simulink model "LinuxMPC"  (Simulink 7.9)
settings: Solver=ode45  StartTime=0.0  StopTime=60  RelTol=1e-3
values from neighbouring files (symbols this model uses):
  P_0 = eye(8)*100    [MPC_setup.m]
  R1 = sqrtm(R)    [MPC_setup.m]
  Ts_control = 0.02    [MPC_setup.m]
  Ts_kalman = 0.01    [MPC_setup.m]
  x_0 = [0,-pi/4,0,0,0,0,0,0]    [MPC_setup.m]
libraries: simulink x3
settings Model: Creator=tna13skn  LastModifiedBy=tna13skn

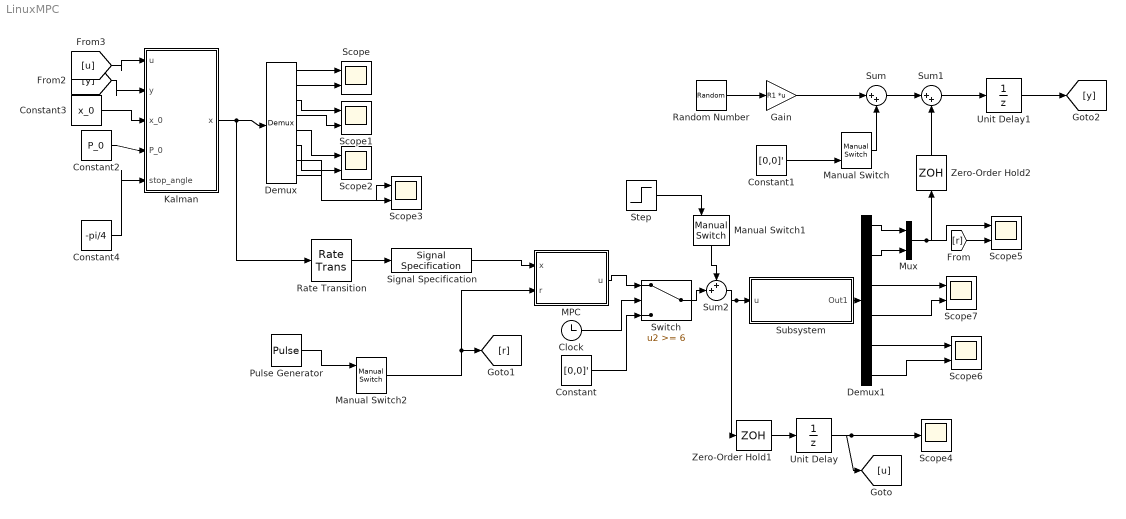
== system LinuxMPC ==
  Clock : Clock
  Constant : Constant  Value=[0,0]'
  Constant1 : Constant  Value=[0,0]'
  Constant2 : Constant  Value=P_0  VectorParams1D=off  SampleTime=Ts_kalman
  Constant3 : Constant  Value=x_0  SampleTime=Ts_kalman
  Constant4 : Constant  Value=-pi/4  SampleTime=Ts_kalman
  Demux : Demux  Outputs=8
  Demux1 : Demux  Outputs=6
  Gain : Gain  Gain=R1  Multiplication=Matrix(K*u)
  Kalman : MATLAB Function  TreatAsAtomicUnit=on
  MPC : MATLAB Function  TreatAsAtomicUnit=on
  Manual Switch : simulink/Signal Routing/Manual Switch  sw=1  action=0  varsize=off
  Manual Switch1 : simulink/Signal Routing/Manual Switch  sw=0  action=0  varsize=off
  Manual Switch2 : simulink/Signal Routing/Manual Switch  sw=1  action=0  varsize=off
  Mux : Mux  Inputs=2
  Pulse Generator : DiscretePulseGenerator  Amplitude=[0,-pi/7]'  Period=20/Ts_control  PulseWidth=10/Ts_control  SampleTime=Ts_control
  Random Number : RandomNumber  Mean=[0,0]'  Variance=[1,1]'  Seed=[1,3]  SampleTime=Ts_kalman
  Rate Transition : RateTransition  X0=x_0  OutPortSampleTime=Ts_control
  Scope{,1..3,5..7} (7 alike) : Scope  NumInputPorts=2
      Scope settings: YMin=-5~-5  YMax=5~5
      Scope1 settings: YMin=-5~-5  YMax=5~5
      Scope2 settings: YMin=-5~-5  YMax=5~5  SaveName=ScopeData2
      Scope3 settings: YMin=-5~-5  YMax=5~5  SaveName=ScopeData3
      Scope5 settings: YMin=-0.8~-0.45  YMax=0.1~0  SaveName=ScopeData5
      Scope6 settings: YMin=-5~-5  YMax=5~5  SaveName=ScopeData6
      Scope7 settings: YMin=-5~-5  YMax=5~5  SaveName=ScopeData7
  Scope4 : Scope
      settings: SaveName=ScopeData4
  Signal Specification : SignalSpecification  Dimensions=[8,1]  SampleTime=Ts_control
      settings: LockScale=on
  Step : Step  Time=30  Before=[0,0]'  After=[1,1]'*0.3  SampleTime=0
  Subsystem : Subsystem
  Sum : Sum  Inputs=|++
  Sum1 : Sum  Inputs=|++
  Sum2 : Sum  Inputs=++|
  Switch : Switch  Threshold=6
  Unit Delay : UnitDelay  SampleTime=-1
  Unit Delay1 : UnitDelay  SampleTime=-1
  Zero-Order Hold1 : ZeroOrderHold  SampleTime=Ts_kalman
  Zero-Order Hold2 : ZeroOrderHold  SampleTime=Ts_kalman
  wires:
  Kalman/1(x) -> Demux/1, Rate Transition/1
  Demux/1 -> Scope/1
  Demux/2 -> Scope/2
  Demux/3 -> Scope1/1
  Demux/4 -> Scope1/2
  Demux/5 -> Scope2/1
  Demux/6 -> Scope2/2
  Rate Transition/1 -> Signal Specification/1
  Signal Specification/1 -> MPC/1(x)
  MPC/1(u) -> Switch/1
  Clock/1 -> Switch/2
  Constant/1 -> Switch/3
  Subsystem/1(Out1) -> Demux1/1
  Demux/7 -> Scope3/1
  Demux/8 -> Scope3/2
  Zero-Order Hold1/1 -> Unit Delay/1
  Unit Delay/1 -> Scope4/1, [u]
  Demux1/1 -> Mux/1
  Demux1/2 -> Mux/2
  Mux/1 -> Scope5/1, Zero-Order Hold2/1
  [r] -> Scope5/2
  Demux1/3 -> Scope7/1
  Demux1/4 -> Scope7/2
  Demux1/5 -> Scope6/1
  Demux1/6 -> Scope6/2
  Random Number/1 -> Gain/1
  Constant1/1 -> Manual Switch/2
  Gain/1 -> Sum/1
  Manual Switch/1 -> Sum/2
  Sum1/1 -> Unit Delay1/1
  Sum/1 -> Sum1/1
  Zero-Order Hold2/1 -> Sum1/2
  Sum2/1 -> Subsystem/1(u), Zero-Order Hold1/1
  Manual Switch1/1 -> Sum2/1
  Step/1 -> Manual Switch1/1
  Manual Switch2/1 -> MPC/2(r), [r]
  Unit Delay1/1 -> [y]
  Pulse Generator/1 -> Manual Switch2/1
  Constant2/1 -> Kalman/4(P_0)
  Constant3/1 -> Kalman/3(x_0)
  [y] -> Kalman/2(y)
  [u] -> Kalman/1(u)
  Constant4/1 -> Kalman/5(stop_angle)
  Switch/1 -> Sum2/2

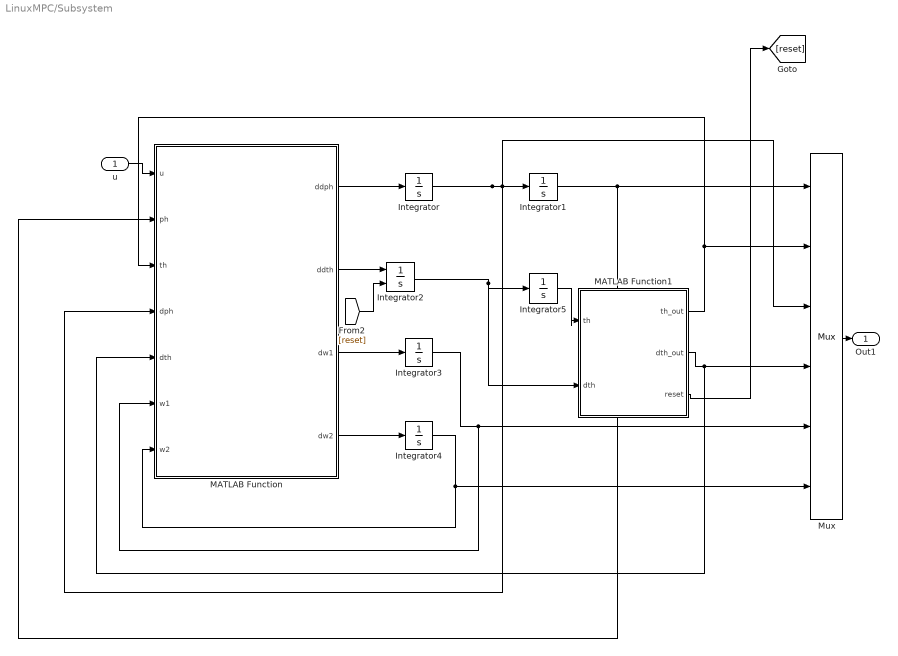
== system LinuxMPC/Subsystem ==
  u : Inport
  Integrator{,1,3..4} (4 alike) : Integrator
  Integrator2 : Integrator  ExternalReset=rising  ShowStatePort=on
  Integrator5 : Integrator  ShowStatePort=on
  MATLAB Function : MATLAB Function  TreatAsAtomicUnit=on
  MATLAB Function1 : MATLAB Function  TreatAsAtomicUnit=on
  Mux : Mux  Inputs=6
  Out1 : Outport
  wires:
  u/1 -> MATLAB Function/1(u)
  MATLAB Function/1(ddph) -> Integrator/1
  Integrator/1 -> Integrator1/1, MATLAB Function/4(dph), Mux/3
  Integrator1/1 -> Mux/1, MATLAB Function/2(ph)
  Mux/1 -> Out1/1
  MATLAB Function/2(ddth) -> Integrator2/1
  MATLAB Function/3(dw1) -> Integrator3/1
  MATLAB Function/4(dw2) -> Integrator4/1
  Integrator4/1 -> Mux/6, MATLAB Function/7(w2)
  Integrator3/1 -> Mux/5, MATLAB Function/6(w1)
  [reset] -> Integrator2/2
  MATLAB Function1/1(th_out) -> Mux/2, MATLAB Function/3(th)
  MATLAB Function1/2(dth_out) -> Mux/4, MATLAB Function/5(dth)
  Integrator5/1 -> MATLAB Function1/1(th)
  Integrator2/1 -> MATLAB Function1/2(dth), Integrator5/1
  MATLAB Function1/3(reset) -> [reset]

== matlab function MPC ==
  data: u output double; x input double; r input double
function u = MPC(x,r)
coder.extrinsic('mycsolve');
u=[0;0];
u=mycsolve(x,r);
end

== matlab function Kalman ==
  data: u input double; y input double; x_0 input double; P_0 input double; stop_angle input double; x output double
function x = kalman(u,y,x_0,P_0,stop_angle)

persistent x_hat;
persistent P;
if(isempty(x_hat))
    x_hat=x_0;
    P=P_0;
end
coder.extrinsic('updateKalman');

[x_hat,P]=updateKalman(x_hat,u,y,P,stop_angle);

x=x_hat;

== matlab function Subsystem/MATLAB Function ==
  data: u input double; ddph output double; ph input double; th input double; dph input double; dth input double; w1 input double; w2 input double; ddth output double; dw1 output double; dw2 output double
function [ddph, ddth, dw1, dw2] = fcn(u, ph, th, dph, dth, w1, w2)
% Implementation of the non-linear integration model derived in the
% technical report "Modelling of the ETH Helicopter Laboratory Process"
% by Magnus Gäfvert, implemented by Marcus Greiff for the project course in
% FRTN01/FRTN15 2018-03-18. The notation and nomenclature vollows the
% report, however, the state vector is defined as
%
%   $x \triangleq [phi; theta; \dot{phi}; \dot{theta}; \omega_1; \omega_2]$
%
% The parameters in Gäfverts report are hard coded in the non-linear model,
% but will be made more general in future revisions.


%% Parameters
% Weights
ml = 0.280;  % [kg]
m1 = 0.3792; % [kg]
m2 = 0.1739; % [kg]
mw = 0.158;  % [kg]
m  = ml + m1 + m2 + mw; % [kg] (eq. 24)

% Distances
l1 = 0.1995; % [m]
l2 = 0.1743; % [m]
lw = 0.090;  % [m]
h  = 0.0298; % [m]
lc = (ml*(l1-l2)+m1*l1-m2*l2-mw*lw)/m; % [m] (eq. 27)

% Inertial parameters
g = 9.81; % [m/s^2]
Ja = 0;   % [] (eq. 26)
Jl = (ml/3)*((l1^3+l2^3)/(l1+l2))+m1*l1^2+m2*l2^2+mw*lw^2; % [] (eq. 25)

% Time, motor and aerodynamics constants
k1 = 1.00e-2; % [Vs/rad]
k2 = 1.39e-2; % [Vs/rad]
C1 = 2.50e-5; % [Ns^/rad^2]
C2 = 1.58e-6; % [Ns^/rad^2]
D1 = 2.90e-7; % [Nms^/rad^2]
D2 = 1.76e-7; % [Nms^/rad^2]
T1 = 1.10;    % [s]
T2 = 0.33;    % [s]


%% Pre-computation of angles and extraction of states
cth = cos(th);
sth = sin(th);
u1 = u(1);
u2 = u(2);

%%rotation stop


%% Integration model
ddph = (cth^2*Jl - 2*h*cth*sth*m*lc + h^2*sth^2*m + Ja)\...
       (2*cth*sth*dph*dth*Jl - 2*h*(sth^2-cth^2)*dph*dth*m*lc - ...
	2*h^2*sth*cth*dph*dth*m + D1*w1*abs(w1)*cth + l2*cth*C2*w2*abs(w2));
ddth = (Jl + h^2*m)\...
       (-cth*sth*dph^2*Jl - h*(-sth^2+cth^2)*dph^2*m*lc - g*cth*m*lc ...
	+ h^2*sth*cth*dph^2*m + m*g*h*sth + l1*C1*w1*abs(w1) + D2*w2*abs(w2));
dw1 = -w1/T1 + u1/(k1*T1);
dw2 = -w2/T2 + u2/(k2*T2);

if(th<=-pi/4&&dth<=0&&ddth<0)
    ddth=0;
end

== matlab function Subsystem/MATLAB Function1 ==
  data: th input double; th_out output double; dth input double; dth_out output double; reset output double
function [th_out,dth_out,reset] = fcn(th,dth)

if(th<=-pi/4&&dth<0)
    th_out=-pi/4;
    dth_out=0;
    reset=1;
    
else
    th_out=th;
    dth_out=dth; 
    reset=0;
end
